simulink model "randamentulpompei"  (R2023b)
settings: Solver=VariableStepAuto  StartTime=0.0  StopTime=10.0  RelTol=1e-3
values from neighbouring files (symbols this model uses):
  keta = 8*10^(-5)    (= 8e-05)    [untitled2.m]
settings Model: Creator=diana.forrai  LastModifiedBy=diana.forrai

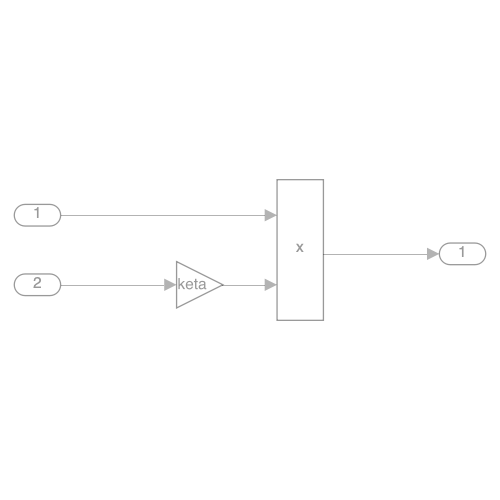
[thumbnail: Simulink's stored preview of the top-level diagram]
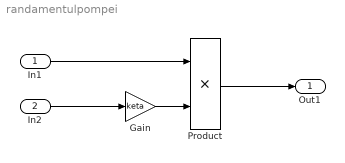
== system randamentulpompei ==
  In1 : Inport
  In2 : Inport  Port=2
  Gain : Gain  Gain=keta
  Product : Product
  Out1 : Outport
  wires:
  Product/1 -> Out1/1
  Gain/1 -> Product/2
  In1/1 -> Product/1
  In2/1 -> Gain/1
